simulink model "StrapDownSim"  (R2013a)
settings: Solver=ode45  StartTime=0.0  StopTime=20  RelTol=1e-3
libraries: simulink x3
settings Model: Creator=Administrator  LastModifiedBy=Administrator

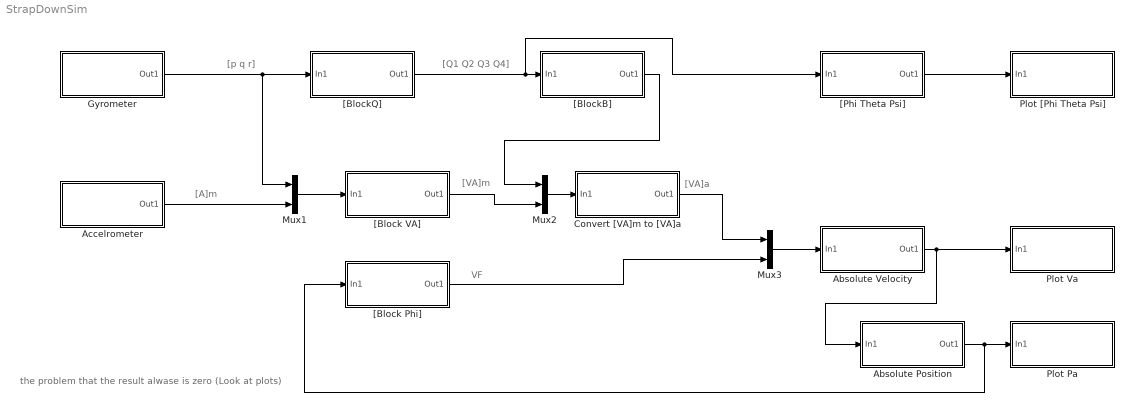
== system StrapDownSim ==
  note: the problem that
      | the result alwase is zero
      | (Look at plots)
  note: [VA]a
  note: [VA]m
  note: VF
  note: [A]m
  note: [Q1 Q2 Q3 Q4]
  note: [p q r]
  Absolute Position : Subsystem
  Absolute Velocity : Subsystem
  Accelrometer : Subsystem
  Convert [VA]m to [VA]a : Subsystem  TreatAsAtomicUnit=on
  Gyrometer : Subsystem
  Mux1 : Mux  Inputs=2
  Mux2 : Mux  Inputs=2
  Mux3 : Mux  Inputs=2
  "Plot Pa " : Subsystem  TreatAsAtomicUnit=on
  Plot Va : Subsystem  TreatAsAtomicUnit=on
  Plot [Phi Theta Psi] : Subsystem  TreatAsAtomicUnit=on
  "[Block Phi]" : Subsystem  TreatAsAtomicUnit=on
  "[Block VA]" : Subsystem  TreatAsAtomicUnit=on
  "[BlockB]" : Subsystem  TreatAsAtomicUnit=on
  "[BlockQ]" : Subsystem  TreatAsAtomicUnit=on
  "[Phi Theta Psi]" : Subsystem  TreatAsAtomicUnit=on
  wires:
  Gyrometer/1(Out1) -> Mux1/1, "[BlockQ]"/1(In1)
  "[BlockB]"/1(Out1) -> Mux2/1
  "[BlockQ]"/1(Out1) -> "[Phi Theta Psi]"/1(In1), "[BlockB]"/1(In1)
  Mux1/1 -> "[Block VA]"/1(In1)
  "[Block VA]"/1(Out1) -> Mux2/2
  "[Block Phi]"/1(Out1) -> Mux3/2
  Mux2/1 -> Convert [VA]m to [VA]a/1(In1)
  Convert [VA]m to [VA]a/1(Out1) -> Mux3/1
  Mux3/1 -> Absolute Velocity/1(In1)
  Absolute Velocity/1(Out1) -> Plot Va/1(In1), Absolute Position/1(In1)
  "[Phi Theta Psi]"/1(Out1) -> Plot [Phi Theta Psi]/1(In1)
  Absolute Position/1(Out1) -> "[Block Phi]"/1(In1), "Plot Pa "/1(In1)
  Accelrometer/1(Out1) -> Mux1/2

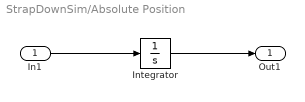
== system StrapDownSim/Absolute Position ==
  In1 : Inport
  Integrator : Integrator
  Out1 : Outport
  wires:
  In1/1 -> Integrator/1
  Integrator/1 -> Out1/1

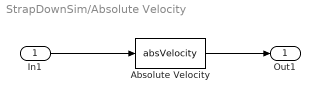
== system StrapDownSim/Absolute Velocity ==
  In1 : Inport
  Absolute Velocity : MATLABFcn  MATLABFcn=absVelocity  OutputDimensions=3
  Out1 : Outport
  wires:
  In1/1 -> Absolute Velocity/1
  Absolute Velocity/1 -> Out1/1

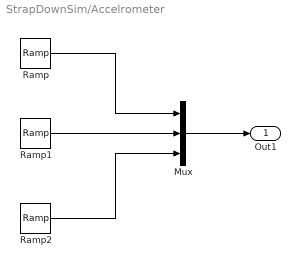
== system StrapDownSim/Accelrometer ==
  Mux : Mux  Inputs=3
  Ramp : simulink/Sources/Ramp  slope=12  start=0  X0=0
  Ramp1 : simulink/Sources/Ramp  slope=0  start=0  X0=0
  Ramp2 : simulink/Sources/Ramp  slope=0  start=0  X0=0
  Out1 : Outport
  wires:
  Mux/1 -> Out1/1
  Ramp1/1 -> Mux/2
  Ramp/1 -> Mux/1
  Ramp2/1 -> Mux/3

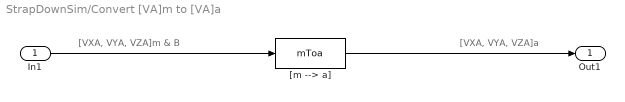
== system StrapDownSim/Convert [VA]m to [VA]a ==
  note: [VXA, VYA, VZA]m & B
  note: [VXA, VYA, VZA]a
  In1 : Inport
  "[m --> a]" : MATLABFcn  MATLABFcn=mToa  OutputDimensions=3
  Out1 : Outport
  wires:
  In1/1 -> "[m --> a]"/1
  "[m --> a]"/1 -> Out1/1

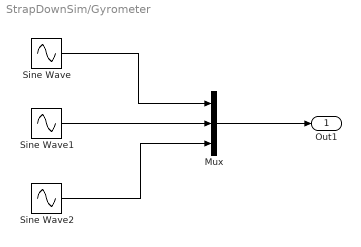
== system StrapDownSim/Gyrometer ==
  Mux : Mux  Inputs=3
  Sine Wave : Sin  Amplitude=2  Frequency=10  SampleTime=0
  Sine Wave1 : Sin  Amplitude=2  Frequency=10  SampleTime=0
  Sine Wave2 : Sin  Amplitude=2  Frequency=10  SampleTime=0
  Out1 : Outport
  wires:
  Mux/1 -> Out1/1
  Sine Wave1/1 -> Mux/2
  Sine Wave/1 -> Mux/1
  Sine Wave2/1 -> Mux/3

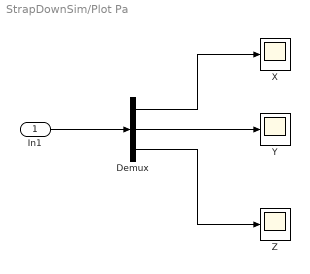
== system StrapDownSim/Plot Pa  ==
  In1 : Inport
  Demux : Demux  Outputs=3
  X : Scope
  Y : Scope
      settings: SaveName=ScopeData3
  Z : Scope
      settings: SaveName=ScopeData4
  wires:
  In1/1 -> Demux/1
  Demux/1 -> X/1
  Demux/2 -> Y/1
  Demux/3 -> Z/1

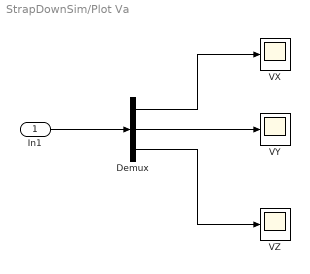
== system StrapDownSim/Plot Va ==
  In1 : Inport
  Demux : Demux  Outputs=3
  VX : Scope
  VY : Scope
      settings: SaveName=ScopeData3
  VZ : Scope
      settings: SaveName=ScopeData4
  wires:
  In1/1 -> Demux/1
  Demux/1 -> VX/1
  Demux/2 -> VY/1
  Demux/3 -> VZ/1

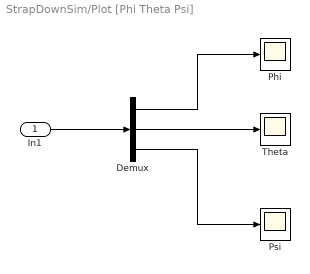
== system StrapDownSim/Plot [Phi Theta Psi] ==
  In1 : Inport
  Demux : Demux  Outputs=3
  Phi : Scope
  Psi : Scope
      settings: SaveName=ScopeData4
  Theta : Scope
      settings: SaveName=ScopeData3
  wires:
  In1/1 -> Demux/1
  Demux/1 -> Phi/1
  Demux/2 -> Theta/1
  Demux/3 -> Psi/1

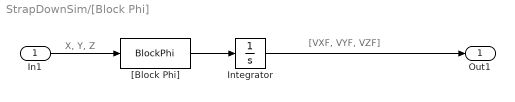
== system StrapDownSim/[Block Phi] ==
  note: X, Y, Z
  note: [VXF, VYF, VZF]
  In1 : Inport
  Integrator : Integrator
  "[Block Phi]" : MATLABFcn  MATLABFcn=BlockPhi  OutputDimensions=3
  Out1 : Outport
  wires:
  "[Block Phi]"/1 -> Integrator/1
  Integrator/1 -> Out1/1
  In1/1 -> "[Block Phi]"/1

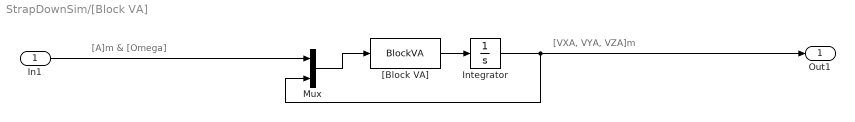
== system StrapDownSim/[Block VA] ==
  note: [A]m & [Omega]
  note: [VXA, VYA, VZA]m
  In1 : Inport
  Integrator : Integrator
  Mux : Mux  Inputs=2
  "[Block VA]" : MATLABFcn  MATLABFcn=BlockVA  OutputDimensions=3
  Out1 : Outport
  wires:
  In1/1 -> Mux/1
  "[Block VA]"/1 -> Integrator/1
  Mux/1 -> "[Block VA]"/1
  Integrator/1 -> Out1/1, Mux/2

== system StrapDownSim/[BlockB] ==
  note: [Q1 Q2 Q3 Q4]
  note: [B_To Convert from movable to absolute ]
  In1 : Inport
  "[Block B]" : MATLABFcn  MATLABFcn=BlockB  OutputDimensions=9
  Out1 : Outport
  wires:
  In1/1 -> "[Block B]"/1
  "[Block B]"/1 -> Out1/1

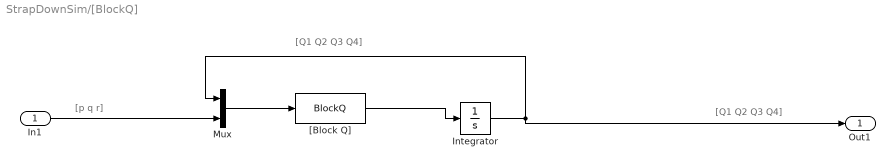
== system StrapDownSim/[BlockQ] ==
  note: [p q r]
  note: [Q1 Q2 Q3 Q4]
  note: [Q1 Q2 Q3 Q4]
  In1 : Inport
  Integrator : Integrator
  Mux : Mux  Inputs=2
  "[Block Q]" : MATLABFcn  MATLABFcn=BlockQ  OutputDimensions=4
  Out1 : Outport
  wires:
  "[Block Q]"/1 -> Integrator/1
  Integrator/1 -> Mux/1, Out1/1
  Mux/1 -> "[Block Q]"/1
  In1/1 -> Mux/2

== system StrapDownSim/[Phi Theta Psi] ==
  note: [B]
  note: [Phi Theta Psi ]
  In1 : Inport
  "[phiTpsi]" : MATLABFcn  MATLABFcn=phiTpsi  OutputDimensions=3
  Out1 : Outport
  wires:
  In1/1 -> "[phiTpsi]"/1
  "[phiTpsi]"/1 -> Out1/1
